simulink model "Control_Test"  (R2024b)
settings: Solver=VariableStepAuto  StartTime=0.0  StopTime=60  RelTol=1e-3
settings Model: Creator=ryang  LastModifiedBy=ryang

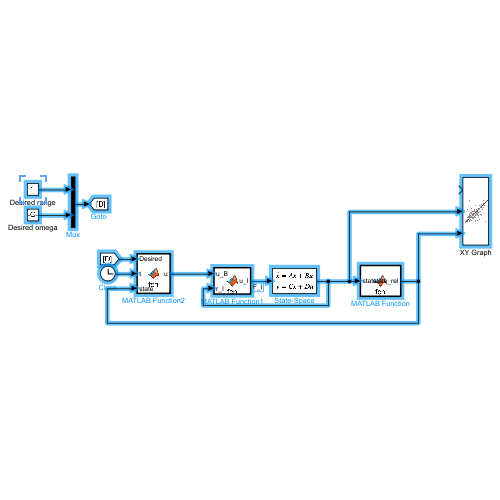
[thumbnail: Simulink's stored preview of the top-level diagram]
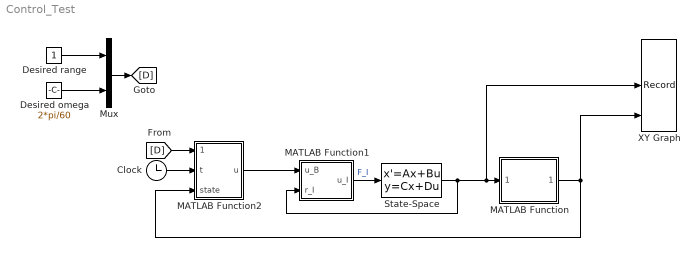
== system Control_Test ==
  Clock : Clock
  Desired omega : Constant  Value=2*pi/60
  Desired range : Constant
  MATLAB Function : MATLAB Function  TreatAsAtomicUnit=on
  MATLAB Function1 : MATLAB Function  TreatAsAtomicUnit=on
  MATLAB Function2 : MATLAB Function  TreatAsAtomicUnit=on
  Mux : Mux  Inputs=2
  State-Space : StateSpace  A=[zeros(3), eye(3); zeros(3,6)]  B=[zeros(3); eye(3)]  C=eye(6)  D=zeros(6,3)  InitialCondition=[-1;0;0;0;0;0]
  XY Graph : Record  FileSettingsInternal="{\"entries\":[{\"content\":{\"excelSettings\":{\"content\":{},\"type\":\"Streamout.ExcelSettings\"}},\"type\":\"Streamout.FileSettingStorage\",\"uuid\":\"\"}],\"packageUris\":[\"http:\\/\\/schema.mathworks.com\\/mf0\\/streamout_blocks\\/R2020a\"],\"version\":\"1.0\"}"  Layout=[1 1]  SignalsInternal="{\"entries\":[{\"content\":{\"signals\":[{\"content\":{\"blockPath\":[],\"dimensions\":[6,1],\"domain\":\"\",\"hasChildren\":true,\"lineColor\":\"#ff13a6\",\"lineWidth\":2,\"port\":2,\"sid\":[\"\"],\"signalID\":1,\"signalName\":\"State-Space\"},\"type\":\"RecordBlkView.Signal\",\"uuid\":\"\"},{\"content\":{\"blockPath\":[],\"channel\":[1,1],\"dimensions\":[6,1],\"domain\":\"\",\"lineColor\":\"#d95319\",\"lineWidth\":2,\"parentID\":1,\"plots\":[ 1 ],\"port\":2,\"sid\":[\"\"],\"signalID\":2,\"signalName\":\"State-Space\"},\"type\":\"RecordBlkView.Signal\",\"uuid\":\"\"},{\"content\":{\"blockPath\":[],\"dimensions\":[6,1],\"domain\":\"\",\"hasChildren\":true,\"lineColor\":\"#22b573\",\"lineWidth\":2,\"port\":3,\"sid\":[\"\"],\"signalID\":3,\"signalName\":\"MATLAB Function\"},\"type\":\"RecordBlkView.Signal\",\"uuid\":\"\"},{\"content\":{\"blockPath\":[],\"channel\":[1,1],\"dimensions\":[6,1],\"domain\":\"\",\"lineColor\":\"#edb120\",\"lineWidth\":2,\"parentID\":3,\"port\":3,\"sid\":[\"\"],\"signalID\":4,\"signalName\":\"MATLAB Function\"},\"type\":\"RecordBlkView.Signal\",\"uuid\":\"\"},{\"content\":{\"blockPath\":[],\"dimensions\":[1],\"domain\":\"\",\"lineColor\":\"#edb120\",\"lineWidth\":2,\"port\":1,\"sid\":[\"\"],\"signalID\":5},\"type\":\"RecordBlkView.Signal\",\"uuid\":\"\"},{\"content\":{\"blockPath\":[],\"channel\":[2,1],\"dimensions\":[6,1],\"domain\":\"\",\"lineColor\":\"#139fff\",\"lineWidth\":2,\"parentID\":1,\"plots\":[ 1 ],\"port\":2,\"sid\":[\"\"],\"signalID\":6,\"signalName\":\"State-Space\"},\"type\":\"RecordBlkView.Signal\",\"uuid\":\"\"},{\"content\":{\"blockPath\":[],\"channel\":[3,1],\"dimensions\":[6,1],\"domain\":\"\",\"lineColor\":\"#ff6929\",\"lineWidth\":2,\"parentID\":1,\"port\":2,\"sid\":[\"\"],\"signalID\":7,\"signalName\":\"State-Space\"},\"type\":\"RecordBlkView.Signal\",\"uuid\":\"\"},{\"content\":{\"blockPath\":[],\"channel\":[4,1],\"dimensions\":[6,1],\"domain\":\"\",\"lineColor\":\"#b746ff\",\"lineWidth\":2,\"parentID\":1,\"port\":2,\"sid\":[\"\"],\"signalID\":8,\"signalName\":\"State-Space\"},\"type\":\"RecordBlkView.Signal\",\"uuid\":\"\"},{\"content\":{\"blockPath\":[],\"channel\":[5,1],\"dimensions\":[6,1],\"domain\":\"\",\"lineColor\":\"#64d413\",\"lineWidth\":2,\"parentID\":1,\"port\":2,\"sid\":[\"\"],\"signalID\":9,\"signalName\":\"State-Space\"},\"type\":\"RecordBlkView.Signal\",\"uuid\":\"\"},{\"content\":{\"blockPath\":[],\"channel\":[6,1],\"dimensions\":[6,1],\"domain\":\"\",\"lineColor\":\"#ff13a6\",\"lineWidth\":2,\"parentID\":1,\"port\":2,\"sid\":[\"\"],\"signalID\":10,\"signalName\":\"State-Space\"},\"type\":\"RecordBlkView.Signal\",\"uuid\":\"\"}]},\"type\":\"RecordBlkView.InputSignals\",\"uuid\":\"\"}],\"packageUris\":[\"http:\\/\\/schema.mathworks.com\\/mf0\\/streamout_blocks\\/R2020a\"],\"version\":\"1.0\"}"  VisualizationBindings="{\"xyplotplugin\":{\"info\":[{\"series\":[{\"bindingParametersList\":[],\"seriesID\":0},{\"bindingParametersList\":[{\"parameter\":\"X-Axis\",\"signalID\":2,\"signalName\":\"State-Space(1,1)\"},{\"parameter\":\"Y-Axis\",\"signalID\":6,\"signalName\":\"State-Space(2,1)\"}],\"seriesID\":1}],\"subplotID\":1}]}}"  CompatibilityTag=XY
  wires:
  State-Space/1 -> XY Graph/2, MATLAB Function/1(state), MATLAB Function1/2(r_I)
  MATLAB Function1/1(u_I) -> State-Space/1  "F_I"
  Desired range/1 -> Mux/1
  Desired omega/1 -> Mux/2
  MATLAB Function2/1(u) -> MATLAB Function1/1(u_B)
  MATLAB Function/1(state_rel) -> XY Graph/3, MATLAB Function2/3(state)
  Mux/1 -> [D]
  [D] -> MATLAB Function2/1(Desired)
  Clock/1 -> MATLAB Function2/2(t)

== matlab function Control_Test/MATLAB Function ==
  data: state input; state_rel output
function state_rel = fcn(state)
% state = [x; y; theta; dx; dy; dtheta]
x   = state(1);
y   = state(2);
th  = state(3);
dx  = state(4);
dy  = state(5);
dth = state(6);

% inertial vector from spacecraft to origin
rI = [-x; -y];

% rotation from inertial -> body
R = [cos(th), sin(th); -sin(th), cos(th)];

% relative position in body
rb = R * rI;        % [r_x; r_y]
r_x = rb(1); r_y = rb(2);

% relative velocity in body
vI = -[dx; dy];          % inertial relative velocity (point is stationary)
Omega = [0, -dth; dth, 0];
vb = R * vI - Omega * rb;  % [v_bx; v_by]

state_rel = [r_x, r_y, th, vb', dth]';

end

% 
% % range and bearing
% rho = norm(rb);
% phi = atan2(r_y, r_x);   % bearing measured in body frame
% range-rate and bearing-rate (guard against rho == 0)
% if rho > 0
%     rho_dot = (rb' * vb) / rho;
%     phi_dot = (r_x * vb(2) - r_y * vb(1)) / (rho^2);
% else
%     rho_dot = 0;
%     phi_dot = 0;
% end

== matlab function Control_Test/MATLAB Function2 ==
  data: Desired input; t input; state input; u output
function u = fcn(Desired, t, state)
% state   = [x_rel; y_rel; theta; dx_rel; dy_rel; dtheta]
% Desired = [x_d; y_d; omega]
% Outputs: [ax_b; ay_b; ath]

    % === Unpack ===
    x_rel = state(1);
    y_rel = state(2);
    th    = state(3);
    dx    = state(4);
    dy    = state(5);
    dth   = state(6);

    x_d   = Desired(1);
    omega = Desired(2);

    % === Gains ===
    kp_xy = 1;   kd_xy = 2;
    kp_th = 1;   kd_th = 5;

    % === Position errors (in inertial frame) ===
    ex  = -x_rel + x_d;
    ey  = -y_rel;
    evx = -dx;
    evy = -dy;

    % === Inertial accelerations from PD ===
    ax_b = kp_xy*ex + kd_xy*evx;
    ay_b = kp_xy*ey + kd_xy*evy;

    % === Attitude control (theta -> ramp) ===
    th_des = omega * t;
    e_th   = wrapToPi(th - th_des);
    e_dth  = dth - omega;

    ath = -kp_th*e_th - kd_th*e_dth;

    % === Output ===
    u = [ax_b; ay_b; ath];
end

== matlab function Control_Test/MATLAB Function1 ==
  data: u_B input; u_I output; r_I input
function u_I = fcn(u_B, r_I)
r_Inert = r_I(3);

s = sin(r_Inert);
c = cos(r_Inert);
R_BI = [c, -s; s, c];

u_I = [-1*R_BI*u_B(1:2); u_B(3)];
